simulink model "l6sim"  (R2022a)
settings: Solver=VariableStepAuto  StartTime=0.0  StopTime=10.0  RelTol=1e-3
values from neighbouring files (symbols this model uses):
  delta_a = 0    [e1516.m]    (also in l6.m)
  delta_y = 0    [l6.m]
  rho = 1    [e1516.m]    (also in l6.m = 0)
  wy = 0    [l6.m]
libraries: cstblocks x2
settings Model: Creator=apple  LastModifiedBy=apple

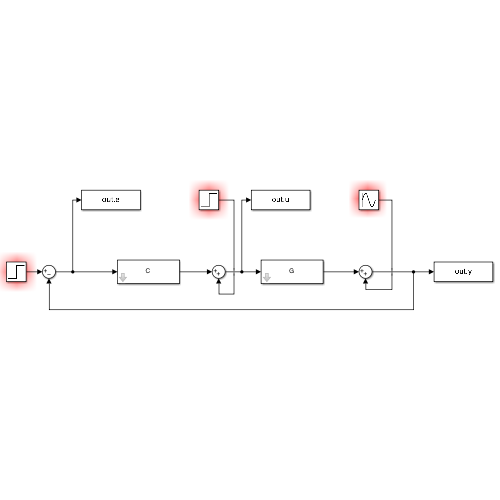
[thumbnail: Simulink's stored preview of the top-level diagram]
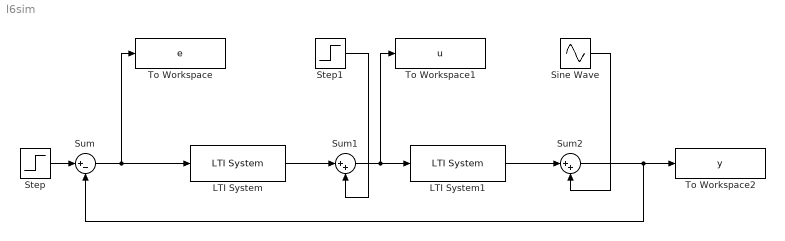
== system l6sim ==
  LTI System : cstblocks/LTI System  sys=C  IC=[]
  LTI System1 : cstblocks/LTI System  sys=G  IC=[]
  Sine Wave : Sin  Amplitude=delta_y  Frequency=wy  SampleTime=0
  Step : Step  Time=0  After=rho  SampleTime=0
  Step1 : Step  Time=0  After=delta_a  SampleTime=0
  Sum : Sum  Inputs=|+-
  Sum1 : Sum  Inputs=|++
  Sum2 : Sum  Inputs=|++
  To Workspace : ToWorkspace  VariableName=e  SaveFormat=Timeseries  SampleTime=-1
  To Workspace1 : ToWorkspace  VariableName=u  SaveFormat=Timeseries  SampleTime=-1
  To Workspace2 : ToWorkspace  VariableName=y  SaveFormat=Timeseries  SampleTime=-1
  wires:
  Step/1 -> Sum/1
  Sum/1 -> To Workspace/1, LTI System/1
  LTI System/1 -> Sum1/1
  Sum1/1 -> To Workspace1/1, LTI System1/1
  Step1/1 -> Sum1/2
  Sine Wave/1 -> Sum2/2
  LTI System1/1 -> Sum2/1
  Sum2/1 -> To Workspace2/1, Sum/2
